simulink model "untitled"  (R2025b)
settings: Solver=VariableStepAuto  StartTime=0.0  StopTime=10.0  RelTol=1e-3
undefined symbols (not defined in the file): DiscIntNeverNeededParam
libraries: simulink x4
settings Model: Creator=mefe  LastModifiedBy=mefe

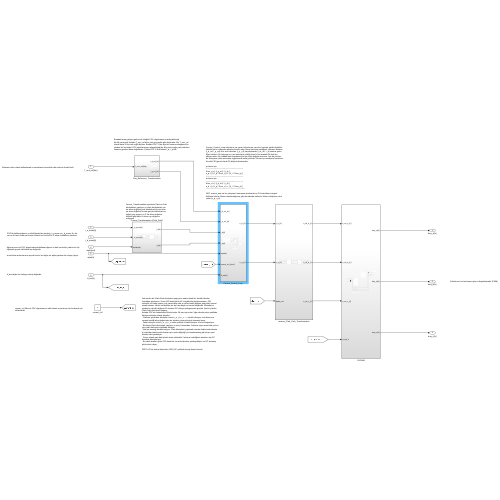
[thumbnail: Simulink's stored preview of the top-level diagram]
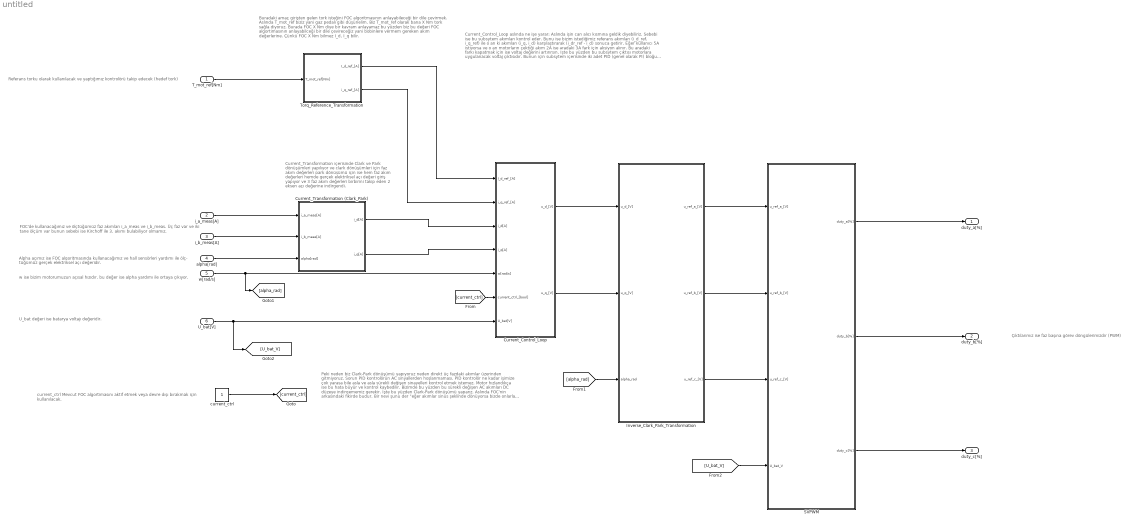
== system untitled ==
  note: Peki neden biz Clark-Park dönüşümü yapıyoruz neden direkt üç fazdaki akımlar üzerinden gitmiyoruz. Sorun PID kontrolörün AC sinyallerden hoşlanmaması. PID kontrolör ne kadar işimize çok yarasa bile asla ve asla sürekli değişen sinayelleri kontrol etmek istemez. Motor hızlandıkça ise bu hata büyür ve kontrol kaybedilir. Bizimde bu yüzden bu sürekli değişen AC akımları DC düzeye indirgememiz gerekir. İşte bu yüzden Clark-Park dönüşümü yaparız.
      | Aslında FOC'nin arkasındaki fikirde budur. Bir nevi şunu der "eğer akımlar sinüs şeklinde dönüyorsa bizde onlarla dönelim".
      | - Statorun gözünden dönüşüm öncesi i_a, i_b, i_c ---> sürekli dönüyor ve kullanıcının vermek istediği akım değerinden bu akımları çıkarıp kontrol etmemiz lazım.
      | - Fakat olmuyor çünkü i_a, i_b, i_c sinüs şeklinde sürekli dönüyor. Kontrol kayboluyor.
      | - İlk olarak Clark dönüşümü yapılıyor ve olay 3 eksenden 2 eksene iniyor ama hala çözüm yok çünkü hala sinüs şeklinde dönüyor.
      | - İşte işin mantığı burada başlıyor. Park dönüşümü yapılarak rotordan bakılıncaki akımlar ile statordan bakılıncaki akımlar aynı anda değiştiği için hareketsizmiş gibi oluyor yani akımlar sabit görünüyor.
      | - Sonuç olarak park dönüşümü sinüs şeklindeki 2 eksene indirdiğimiz akımları alıp DC akımlara dönüştürüyor.
      | - Bu sabit akımları gören PID kontrolör ise artık akımları yakalayabiliyor ve DC akımmış gibi kontrol ediyor.
      |
      | ÖZET: AC bir sistemi kontrolöre (PID) DC şeklinde tanıtıp kontrol etmek.
  note: Current_Control_Loop aslında ne işe yarar: Aslında işin can alıcı kısmına geldik diyebiliriz. Sebebi ise bu subsytem akımları kontrol eder. Bunu ise bizim istediğimiz referans akımları (i_d_ref, i_q_ref) ile o an ki akımları (i_q, i_d) karşılaştırarak (i_dr_ref - i_d) sonuca getirir. Eğer kullanıcı 5A istiyorsa ve o an motorların çektiği akım 2A ise aradaki 3A fark için aksiyon alınır. Bu aradaki farkı kapatmak için ise voltaj değerini artırırsın. İşte bu yüzden bu subsytem çıktısı motorlara uygulanacak voltaj çıktısıdır. Bunun için subsytem içerisinde iki adet PID (genel olarak PI) bloğu kullanılacaktır.
      |
      | q ekseni için
      | ----------------------------------------------------------
      | Error_q = [ (i_q_ref) - (i_q) ]
      | u_q = [ ( K_p * Error_q ) + ( K_i * Error_q ) ]
      | ----------------------------------------------------------
      | d ekseni için
      | ----------------------------------------------------------
      | Error_d = [ (i_d_ref) - (i_d) ]
      | u_d = [ ( K_p * Error_d ) + ( K_i * Error_d ) ]
      | -------------------------------------------------------------
      |
      | NOT: current_ena ise bu subsytem'i tamamen durdurmak ve PI kontrolünün integral birikimini sıfırlar. Motoru durdurduğumuz gibi durumlarda kullanılır. Motor voltajlarını sıfıra çeker (u_q, u_d).
  note: Buradaki amaç girişten gelen tork isteğini FOC algoritmasının anlayabileceği
      | bir dile çevirmek. Aslında T_mot_ref biziz yani gaz pedalı gibi düşünelim. Biz T_mot_ref olarak bana X Nm tork sağla diyoruz. Burada FOC X Nm diye bir kavram anlayamaz bu yüzden biz bu değeri FOC algortimasının anlayabilceği bir dile çevireceğiz yani bobinlere vermem gereken akım değerlerine. Çünkü FOC X Nm bilmez I_d, I_q bilir.
  note: Current_Transformation içerisinde Clark ve Park dönüşümleri yapılıyor ve clark dönüşümleri için faz akım değerleri park dönüşümü için ise hem faz akım değerleri hemde gerçek elektriksel açı değeri giriş yapıyor ve 3 faz akım değerleri birbirini takip eden 2 eksen açı değerine indirgendi.
  note: Çıktılarımız ise faz başına görev döngülerimizdir (PWM)
  note: U_bat değeri ise batarya voltajı değeridir.
  note: current_ctrl Mevcut FOC algortimasını aktif etmek veya devre dışı bırakmak için kullanılacak.
  note: w ise bizim motorumuzun açısal hızıdır. bu değer ise alpha yardımı ile ortaya çıkıyor.
  note: Alpha açımız ise FOC algoritmasında kullanacağımız ve hall sensörleri yardımı ile ölç-
      | tüğümüz gerçek elektriksel açı değeridir.
  note: FOC'de kullanacağımız ve ölçtüğümüz faz akımları i_a_meas ve i_b_meas. Üç faz var ve iki tane ölçüm var bunun sebebi ise Kirchoff ile 3. akımı bulabiliyor olmamız.
  note: Referans torku olarak kullanılacak ve yaptığımız kontrolörü takip edecek (hedef tork)
  T_mot_ref[Nm] : Inport
  i_a_meas[A] : Inport  Port=2
  i_b_meas[A] : Inport  Port=3
  alpha[rad] : Inport  Port=4
  w[rad/s] : Inport  Port=5
  U_bat[V] : Inport  Port=6
  Current_Control_Loop : Subsystem
  Current_Transformation (Clark_Park) : Subsystem
  Inverse_Clark_Park_Transformation : Subsystem
  SVPWM : Subsystem
  Torq_Reference_Transformation : Subsystem
  current_ctrl : Constant
  duty_a[%] : Outport
  duty_b[%] : Outport  Port=2
  duty_c[%] : Outport  Port=3
  wires:
  i_a_meas[A]/1 -> Current_Transformation (Clark_Park)/1(i_a_meas[A])
  i_b_meas[A]/1 -> Current_Transformation (Clark_Park)/2(i_b_meas[A])
  alpha[rad]/1 -> Current_Transformation (Clark_Park)/3(alpha[rad])
  T_mot_ref[Nm]/1 -> Torq_Reference_Transformation/1(T_mot_ref[Nm])
  Torq_Reference_Transformation/1(I_d_ref_[A]) -> Current_Control_Loop/1(I_d_ref_[A])
  Torq_Reference_Transformation/2(i_q_ref_[A]) -> Current_Control_Loop/2(i_q_ref_[A])
  Current_Transformation (Clark_Park)/1(i_d[A]) -> Current_Control_Loop/3(i_d[A])
  Current_Transformation (Clark_Park)/2(i_q[A]) -> Current_Control_Loop/4(i_q[A])
  current_ctrl/1 -> [current_ctrl]
  [current_ctrl] -> Current_Control_Loop/6(current_ctrl_[bool])
  w[rad/s]/1 -> [alpha_rad], Current_Control_Loop/5(w[rad/s])
  U_bat[V]/1 -> [U_bat_V], Current_Control_Loop/7(U_bat[V])
  [alpha_rad] -> Inverse_Clark_Park_Transformation/3(alpha_rad)
  Current_Control_Loop/2(u_q_[V]) -> Inverse_Clark_Park_Transformation/2(u_q_[V])
  Current_Control_Loop/1(u_d_[V]) -> Inverse_Clark_Park_Transformation/1(u_d_[V])
  Inverse_Clark_Park_Transformation/1(u_ref_a_[V]) -> SVPWM/1(u_ref_a_[V])
  Inverse_Clark_Park_Transformation/2(u_ref_b_[V]) -> SVPWM/2(u_ref_b_[V])
  Inverse_Clark_Park_Transformation/3(u_ref_c_[V]) -> SVPWM/3(u_ref_c_[V])
  [U_bat_V] -> SVPWM/4(U_bat_V)
  SVPWM/1(duty_a[%]) -> duty_a[%]/1
  SVPWM/3(duty_c[%]) -> duty_c[%]/1
  SVPWM/2(duty_b[%]) -> duty_b[%]/1

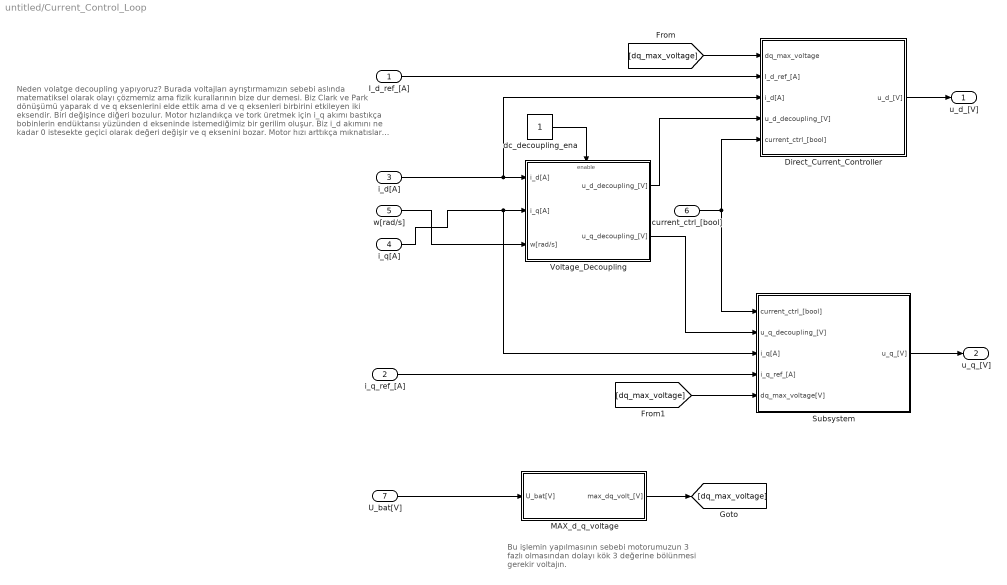
== system untitled/Current_Control_Loop ==
  note: Neden volatge decoupling yapıyoruz? Burada voltajları ayrıştırmamızın sebebi aslında matematiksel olarak olayı çözmemiz ama fizik kurallarının bize dur demesi. Biz Clark ve Park dönüşümü yaparak d ve q eksenlerini elde ettik ama d ve q eksenleri birbirini etkileyen iki eksendir. Biri değişince diğeri bozulur.
      | Motor hızlandıkça ve tork üretmek için i_q akımı bastıkça bobinlerin endüktansı yüzünden d ekseninde istemediğimiz bir gerilim oluşur.
      | Biz i_d akımını ne kadar 0 istesekte geçici olarak değeri değişir ve q eksenini bozar.
      | Motor hızı arttıkça mıknatıslar bobinlerde ters gerilim (Back-EMF) üretir. Bu gerilim doğrudan q eksenindeki voltajı düşürür.
      | NOT: Motor hızlandıkça torkun düşmesinin ana sebebi budur.
      | Peki bu olayların bu yapıya etkisi ne olur?
      | Yapı i_d =0 olsun ister. d ekseni PI kontrolcüsü işini yapmaya çalışır.
      | Yandan kullanıcı gaza basar yani i_q'yu arttırır ve fizik kuralları gereği d ekseninde bir dalgalanma olur.
      | Bu durumda PI kontrolcüsü bu hatayı düzeltmeye çalışır ama gecikmeli tepki verir ve kontrolden çıkar.
      |
      | NOT: FOC dögüsünden çıkıp yüksek hızlara giderken (Back-EMF) bu yapı hayat kurtaracak ve prüzsüz geçiş için yardımcı olacak.
  note: Bu işlemin yapılmasının sebebi motorumuzun
      | 3 fazlı olmasından dolayı kök 3 değerine
      | bölünmesi gerekir voltajın.
  I_d_ref_[A] : Inport
  i_q_ref_[A] : Inport  Port=2
  i_d[A] : Inport  Port=3
  i_q[A] : Inport  Port=4
  w[rad/s] : Inport  Port=5
  current_ctrl_[bool] : Inport  Port=6
  U_bat[V] : Inport  Port=7
  Direct_Current_Controller : Subsystem
  MAX_d_q_voltage : Subsystem
  Subsystem : Subsystem
  Voltage_Decoupling : Subsystem
  dc_decoupling_ena : Constant
  u_d_[V] : Outport
  u_q_[V] : Outport  Port=2
  wires:
  w[rad/s]/1 -> Voltage_Decoupling/3(w[rad/s])
  i_d[A]/1 -> Voltage_Decoupling/1(i_d[A]), Direct_Current_Controller/3(i_d[A])
  i_q[A]/1 -> Subsystem/3(i_q[A]), Voltage_Decoupling/2(i_q[A])
  I_d_ref_[A]/1 -> Direct_Current_Controller/2(I_d_ref_[A])
  Voltage_Decoupling/1(u_d_decoupling_[V]) -> Direct_Current_Controller/4(u_d_decoupling_[V])
  Direct_Current_Controller/1(u_d_[V]) -> u_d_[V]/1
  current_ctrl_[bool]/1 -> Subsystem/1(current_ctrl_[bool]), Direct_Current_Controller/5(current_ctrl_[bool])
  U_bat[V]/1 -> MAX_d_q_voltage/1(U_bat[V])
  MAX_d_q_voltage/1(max_dq_volt_[V]) -> [dq_max_voltage]
  [dq_max_voltage] -> Direct_Current_Controller/1(dq_max_voltage)
  Subsystem/1(u_q_[V]) -> u_q_[V]/1
  Voltage_Decoupling/2(u_q_decoupling_[V]) -> Subsystem/2(u_q_decoupling_[V])
  i_q_ref_[A]/1 -> Subsystem/4(i_q_ref_[A])
  [dq_max_voltage] -> Subsystem/5(dq_max_voltage[V])
  dc_decoupling_ena/1 -> Voltage_Decoupling/Enable

== system untitled/Current_Transformation (Clark_Park) ==
  i_a_meas[A] : Inport
  i_b_meas[A] : Inport  Port=2
  alpha[rad] : Inport  Port=3
  Clark_Transformation : Subsystem
  Park_Transformation : Subsystem
  i_d[A] : Outport
  i_q[A] : Outport  Port=2
  wires:
  i_a_meas[A]/1 -> Clark_Transformation/1(i_a_meas[A])
  i_b_meas[A]/1 -> Clark_Transformation/2(i_b_meas[A])
  Clark_Transformation/1(i_x[A]) -> Park_Transformation/1(i_x[A])  "i_x_meas"
  Clark_Transformation/2(i_y[A]) -> Park_Transformation/2(i_y[A])  "i_y_meas"
  alpha[rad]/1 -> Park_Transformation/3(alpha[rad])
  Park_Transformation/1(i_d[A]) -> i_d[A]/1  "i_d_meas"
  Park_Transformation/2(i_q[A]) -> i_q[A]/1  "i_q_meas"

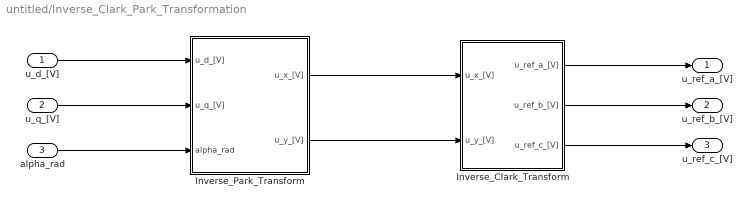
== system untitled/Inverse_Clark_Park_Transformation ==
  u_d_[V] : Inport
  u_q_[V] : Inport  Port=2
  alpha_rad : Inport  Port=3
  Inverse_Clark_Transform : Subsystem
  Inverse_Park_Transform : Subsystem
  u_ref_a_[V] : Outport
  u_ref_b_[V] : Outport  Port=2
  u_ref_c_[V] : Outport  Port=3
  wires:
  u_d_[V]/1 -> Inverse_Park_Transform/1(u_d_[V])
  u_q_[V]/1 -> Inverse_Park_Transform/2(u_q_[V])
  alpha_rad/1 -> Inverse_Park_Transform/3(alpha_rad)
  Inverse_Clark_Transform/1(u_ref_a_[V]) -> u_ref_a_[V]/1
  Inverse_Clark_Transform/3(u_ref_c_[V]) -> u_ref_c_[V]/1
  Inverse_Clark_Transform/2(u_ref_b_[V]) -> u_ref_b_[V]/1
  Inverse_Park_Transform/1(u_x_[V]) -> Inverse_Clark_Transform/1(u_x_[V])
  Inverse_Park_Transform/2(u_y_[V]) -> Inverse_Clark_Transform/2(u_y_[V])

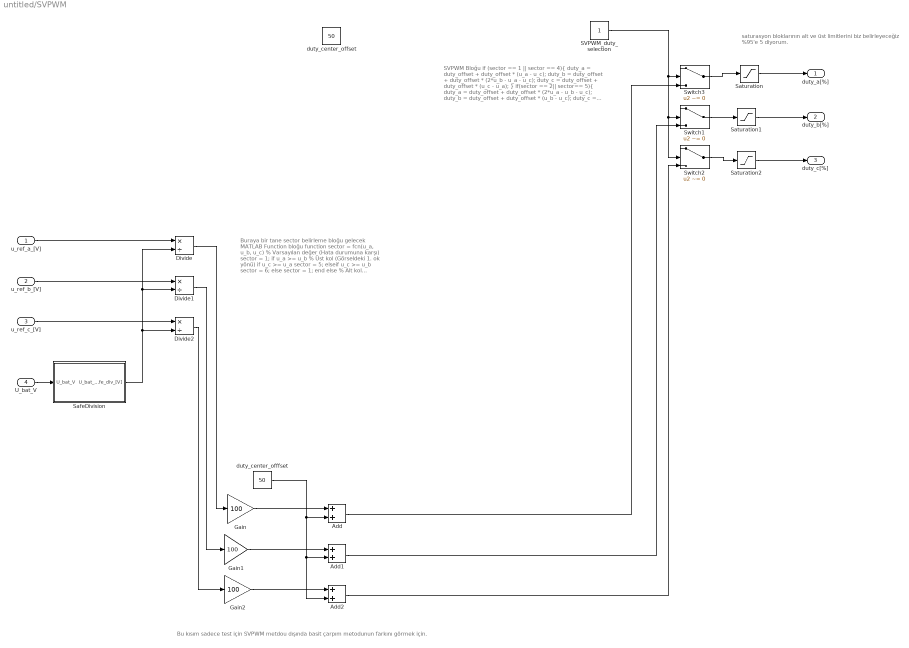
== system untitled/SVPWM ==
  note: saturasyon bloklarının alt ve üst limitlerini biz belirleyeceğiz
      | %95'e 5 diyorum.
  note: Bu kısım sadece test için SVPWM metdou dışında basit çarpım metodunun farkını görmek için.
  note: SVPWM Bloğu
      |
      | if (sector == 1 || sector == 4){
      | duty_a = duty_offset + duty_offset * (u_a - u_c);
      | duty_b = duty_offset + duty_offset * (2*u_b - u_a - u_c);
      | duty_c = duty_offset + duty_offset * (u_c - u_a);
      | }
      | if(sector == 2|| sector== 5){
      | duty_a = duty_offset + duty_offset * (2*u_a - u_b - u_c);
      | duty_b = duty_offset + duty_offset * (u_b - u_c);
      | duty_c = duty_offset + duty_offset * (u_c - u_b);
      | }
      | if(sector == 3 || sector == 6){
      | duty_c = duty_offset + duty_offset * (u_a - u_b);
      | duty_c = duty_offset + duty_offset * (u_b - u_a);
      | duty_a = duty_offset + duty_offset * (2*u_c - u_a - u_b);
      | }
  note: Buraya bir tane sector belirleme
      | bloğu gelecek
      | MATLAB Function bloğu
      | function sector = fcn(u_a, u_b, u_c)
      |     % Varsayılan değer (Hata durumuna karşı)
      |     sector = 1;
      |
      |     if u_a >= u_b
      |         % Üst kol (Görseldeki 1. ok yönü)
      |         if u_c >= u_a
      |             sector = 5;
      |         elseif u_c >= u_b
      |             sector = 6;
      |         else
      |             sector = 1;
      |         end
      |     else
      |         % Alt kol (Görseldeki 2. ok yönü: u_a < u_b)
      |         if u_c >= u_b
      |             sector = 2;
      |         elseif u_a >= u_c
      |             sector = 3;
      |         else
      |             sector = 4;
      |         end
      |     end
      | end
  u_ref_a_[V] : Inport
  u_ref_b_[V] : Inport  Port=2
  u_ref_c_[V] : Inport  Port=3
  U_bat_V : Inport  Port=4
  Add : Sum
  Add1 : Sum
  Add2 : Sum
  Divide : Product  Inputs=*/
  Divide1 : Product  Inputs=*/
  Divide2 : Product  Inputs=*/
  Gain : Gain  Gain=100  OutDataTypeStr=single
  Gain1 : Gain  Gain=100  OutDataTypeStr=single
  Gain2 : Gain  Gain=100  OutDataTypeStr=single
  SVPWM_duty_selection : Constant  OutDataTypeStr=boolean
  SafeDivision : Subsystem
  Saturation : Saturate  UpperLimit=95  LowerLimit=5
  Saturation1 : Saturate  UpperLimit=95  LowerLimit=5
  Saturation2 : Saturate  UpperLimit=95  LowerLimit=5
  Switch1 : Switch  Criteria=u2 ~= 0  SaturateOnIntegerOverflow=off  InputSameDT=off
  Switch2 : Switch  Criteria=u2 ~= 0  SaturateOnIntegerOverflow=off  InputSameDT=off
  Switch3 : Switch  Criteria=u2 ~= 0  SaturateOnIntegerOverflow=off  InputSameDT=off
  duty_center_offfset : Constant  Value=50  OutDataTypeStr=single
  duty_center_offset : Constant  Value=50  OutDataTypeStr=single
  duty_a[%] : Outport
  duty_b[%] : Outport  Port=2
  duty_c[%] : Outport  Port=3
  wires:
  U_bat_V/1 -> SafeDivision/1(U_bat_V)
  u_ref_b_[V]/1 -> Divide1/1
  u_ref_a_[V]/1 -> Divide/1
  u_ref_c_[V]/1 -> Divide2/1
  SafeDivision/1(U_bat_safe_div_[V]) -> Divide2/2, Divide1/2, Divide/2
  Gain/1 -> Add/1
  Gain1/1 -> Add1/1
  Gain2/1 -> Add2/1
  Divide2/1 -> Gain2/1
  Divide1/1 -> Gain1/1
  Divide/1 -> Gain/1
  duty_center_offfset/1 -> Add/2, Add2/2, Add1/2
  Add/1 -> Switch3/3
  Add1/1 -> Switch1/3
  Add2/1 -> Switch2/3
  SVPWM_duty_selection/1 -> Switch3/2, Switch1/2, Switch2/2
  Switch3/1 -> Saturation/1
  Switch1/1 -> Saturation1/1
  Switch2/1 -> Saturation2/1
  Saturation2/1 -> duty_c[%]/1
  Saturation1/1 -> duty_b[%]/1
  Saturation/1 -> duty_a[%]/1

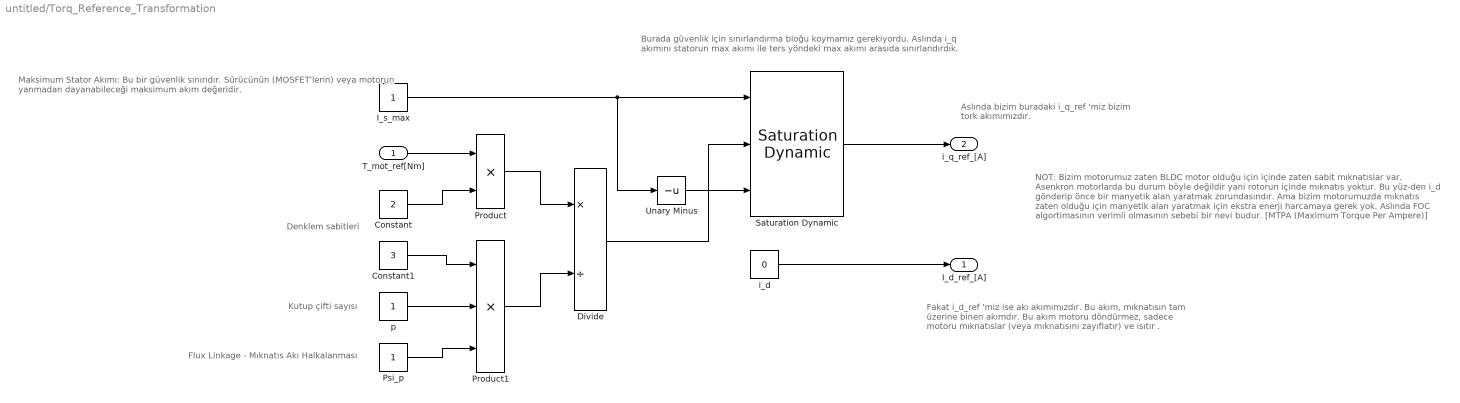
== system untitled/Torq_Reference_Transformation ==
  note: NOT: Bizim motorumuz zaten BLDC motor olduğu için içinde zaten sabit mıknatıslar var.
      | Asenkron motorlarda bu durum böyle değildir yani rotorun içinde mıknatıs yoktur. Bu yüz-den i_d gönderip önce bir manyetik alan yaratmak zorundasındır.
      | Ama bizim motorumuzda mıknatıs zaten olduğu için manyetik alan yaratmak için ekstra
      | enerji harcamaya gerek yok.
      | Aslında FOC algortimasının verimli olmasının sebebi bir nevi budur.
      | [MTPA (Maximum Torque Per Ampere)]
  note: Fakat i_d_ref 'miz ise akı akımımızdır.
      | Bu akım, mıknatısın tam üzerine binen akımdır.
      | Bu akım motoru döndürmez, sadece motoru mıknatıslar
      | (veya mıknatısını zayıflatır) ve ısıtır .
  note: Aslında bizim buradaki i_q_ref 'miz bizim
      | tork akımımızdır.
  note: Denklem sabitleri
  note: Burada güvenlik için sınırlandırma bloğu koymamız gerekiyordu. Aslında i_q
      | akımını statorun max akımı ile ters yöndeki max akımı arasıda sınırlandırdık.
  note: Maksimum Stator Akımı: Bu bir güvenlik sınırıdır. Sürücünün (MOSFET'lerin) veya motorun yanmadan dayanabileceği maksimum akım değeridir.
  note: Flux Linkage - Mıknatıs Akı Halkalanması
  note: Kutup çifti sayısı
  T_mot_ref[Nm] : Inport
  Constant : Constant  Value=2  OutDataTypeStr=single
  Constant1 : Constant  Value=3  OutDataTypeStr=single
  Divide : Product  Inputs=*/
  I_s_max : Constant
  Product : Product
  Product1 : Product  Inputs=3
  Psi_p : Constant
  Saturation Dynamic : simulink/Discontinuities/Saturation Dynamic  OutMin=[]  OutMax=[]  OutDataTypeStr=Inherit: Same as second input  OutDataType=fixdt(1, 16)  OutScaling=2^-10  DoSatur=off
  Unary Minus : UnaryMinus
  i_d : Constant  Value=0  OutDataTypeStr=single
  p : Constant
  I_d_ref_[A] : Outport
  i_q_ref_[A] : Outport  Port=2
  wires:
  T_mot_ref[Nm]/1 -> Product/1
  Constant/1 -> Product/2
  Constant1/1 -> Product1/1
  p/1 -> Product1/2
  Psi_p/1 -> Product1/3
  Product/1 -> Divide/1
  Product1/1 -> Divide/2
  I_s_max/1 -> Unary Minus/1, Saturation Dynamic/1
  Unary Minus/1 -> Saturation Dynamic/3
  Divide/1 -> Saturation Dynamic/2
  Saturation Dynamic/1 -> i_q_ref_[A]/1
  i_d/1 -> I_d_ref_[A]/1

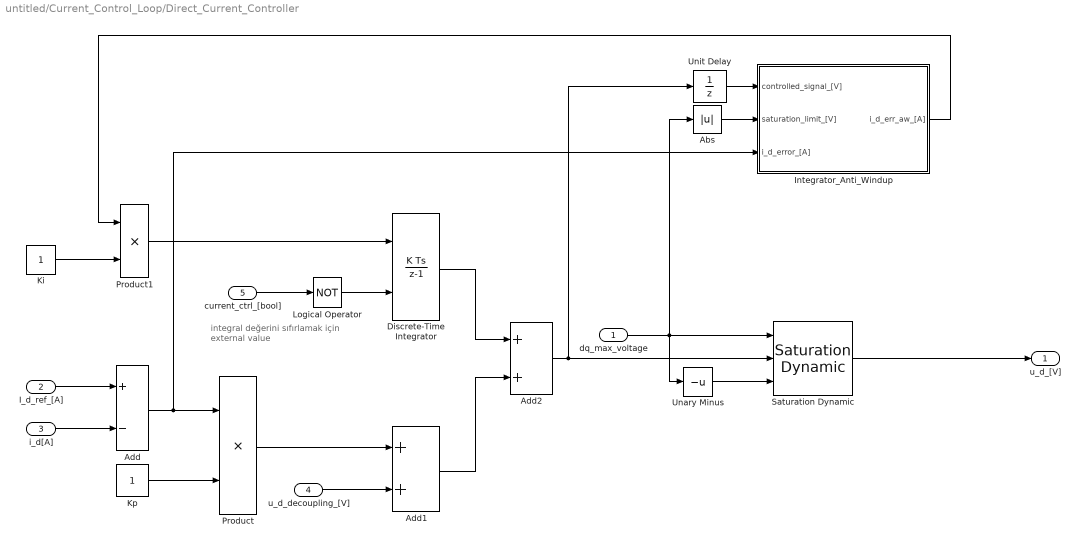
== system untitled/Current_Control_Loop/Direct_Current_Controller ==
  note: integral değerini
      | sıfırlamak için
      | external value
  dq_max_voltage : Inport
  I_d_ref_[A] : Inport  Port=2
  i_d[A] : Inport  Port=3
  u_d_decoupling_[V] : Inport  Port=4
  current_ctrl_[bool] : Inport  Port=5
  Abs : Abs  SaturateOnIntegerOverflow=off
  Add : Sum  Inputs=+-
  Add1 : Sum
  Add2 : Sum
  Discrete-Time Integrator : DiscreteIntegrator  ExternalReset=level  SampleTime=-1  ICPrevOutput=DiscIntNeverNeededParam  ICPrevScaledInput=DiscIntNeverNeededParam
  Integrator_Anti_Windup : Subsystem
  Ki : Constant
  Kp : Constant
  Logical Operator : Logic  Operator=NOT  AllPortsSameDT=off  OutDataTypeStr=boolean
  Product : Product
  Product1 : Product
  Saturation Dynamic : simulink/Discontinuities/Saturation Dynamic  OutMin=[]  OutMax=[]  OutDataTypeStr=Inherit: Same as second input  OutDataType=fixdt(1, 16)  OutScaling=2^-10  DoSatur=off
  Unary Minus : UnaryMinus
  Unit Delay : UnitDelay  SampleTime=-1  HasFrameUpgradeWarning=on
  u_d_[V] : Outport
  wires:
  I_d_ref_[A]/1 -> Add/1
  i_d[A]/1 -> Add/2
  Kp/1 -> Product/2
  Add/1 -> Integrator_Anti_Windup/3(i_d_error_[A]), Product/1
  Product/1 -> Add1/1
  u_d_decoupling_[V]/1 -> Add1/2
  Ki/1 -> Product1/2
  Product1/1 -> Discrete-Time Integrator/1
  current_ctrl_[bool]/1 -> Logical Operator/1
  Logical Operator/1 -> Discrete-Time Integrator/2
  Discrete-Time Integrator/1 -> Add2/1
  Add1/1 -> Add2/2
  Add2/1 -> Unit Delay/1, Saturation Dynamic/2
  Saturation Dynamic/1 -> u_d_[V]/1
  dq_max_voltage/1 -> Abs/1, Unary Minus/1, Saturation Dynamic/1
  Unary Minus/1 -> Saturation Dynamic/3
  Unit Delay/1 -> Integrator_Anti_Windup/1(controlled_signal_[V])
  Integrator_Anti_Windup/1(i_d_err_aw_[A]) -> Product1/1
  Abs/1 -> Integrator_Anti_Windup/2(saturation_limit_[V])

== system untitled/Current_Control_Loop/MAX_d_q_voltage ==
  U_bat[V] : Inport
  1/sqrt(3) (dq_voltage_ratio) : Constant
  Product : Product
  max_dq_volt_[V] : Outport
  wires:
  Product/1 -> max_dq_volt_[V]/1
  U_bat[V]/1 -> Product/1
  1/sqrt(3) (dq_voltage_ratio)/1 -> Product/2

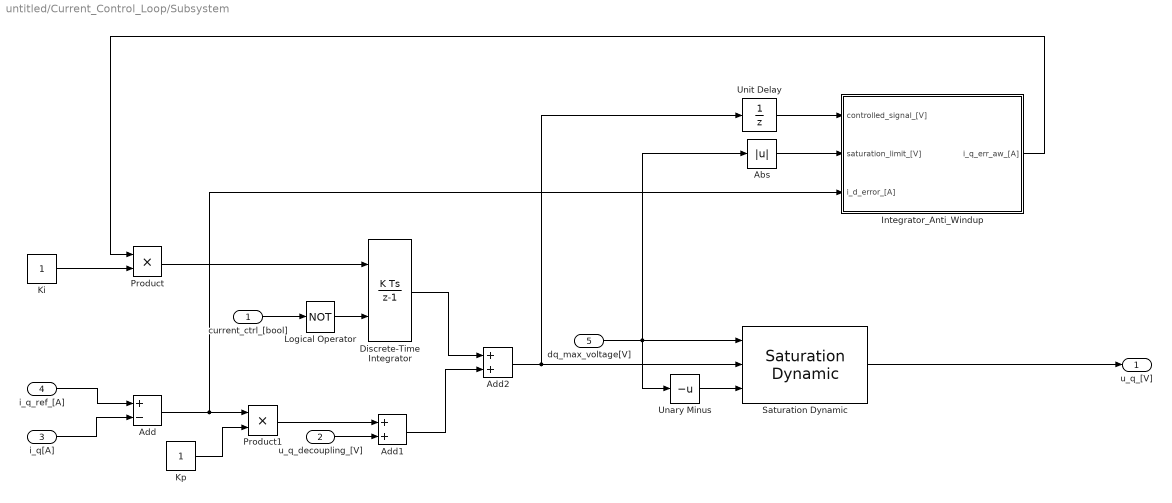
== system untitled/Current_Control_Loop/Subsystem ==
  current_ctrl_[bool] : Inport
  u_q_decoupling_[V] : Inport  Port=2
  i_q[A] : Inport  Port=3
  i_q_ref_[A] : Inport  Port=4
  dq_max_voltage[V] : Inport  Port=5
  Abs : Abs  SaturateOnIntegerOverflow=off
  Add : Sum  Inputs=+-
  Add1 : Sum
  Add2 : Sum
  Discrete-Time Integrator : DiscreteIntegrator  ExternalReset=level  SampleTime=-1  ICPrevOutput=DiscIntNeverNeededParam  ICPrevScaledInput=DiscIntNeverNeededParam
  Integrator_Anti_Windup : Subsystem
  Ki : Constant
  Kp : Constant
  Logical Operator : Logic  Operator=NOT  AllPortsSameDT=off  OutDataTypeStr=boolean
  Product : Product
  Product1 : Product
  Saturation Dynamic : simulink/Discontinuities/Saturation Dynamic  OutMin=[]  OutMax=[]  OutDataTypeStr=Inherit: Same as second input  OutDataType=fixdt(1, 16)  OutScaling=2^-10  DoSatur=off
  Unary Minus : UnaryMinus
  Unit Delay : UnitDelay  SampleTime=-1  HasFrameUpgradeWarning=on
  u_q_[V] : Outport
  wires:
  Unit Delay/1 -> Integrator_Anti_Windup/1(controlled_signal_[V])
  Abs/1 -> Integrator_Anti_Windup/2(saturation_limit_[V])
  Add/1 -> Integrator_Anti_Windup/3(i_d_error_[A]), Product1/1
  Integrator_Anti_Windup/1(i_q_err_aw_[A]) -> Product/1
  Ki/1 -> Product/2
  Kp/1 -> Product1/2
  i_q_ref_[A]/1 -> Add/1
  i_q[A]/1 -> Add/2
  Logical Operator/1 -> Discrete-Time Integrator/2
  current_ctrl_[bool]/1 -> Logical Operator/1
  Product/1 -> Discrete-Time Integrator/1
  Product1/1 -> Add1/1
  u_q_decoupling_[V]/1 -> Add1/2
  Discrete-Time Integrator/1 -> Add2/1
  Add1/1 -> Add2/2
  Add2/1 -> Saturation Dynamic/2, Unit Delay/1
  dq_max_voltage[V]/1 -> Abs/1, Unary Minus/1, Saturation Dynamic/1
  Unary Minus/1 -> Saturation Dynamic/3
  Saturation Dynamic/1 -> u_q_[V]/1

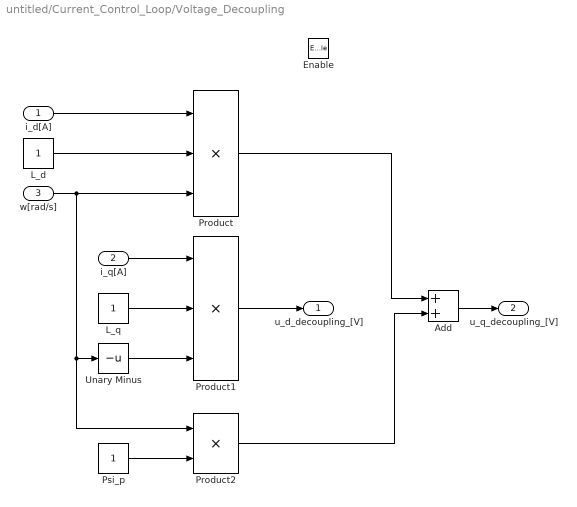
== system untitled/Current_Control_Loop/Voltage_Decoupling ==
  i_d[A] : Inport
  i_q[A] : Inport  Port=2
  w[rad/s] : Inport  Port=3
  Enable : EnablePort
  Add : Sum
  L_d : Constant
  L_q : Constant
  Product : Product  Inputs=3
  Product1 : Product  Inputs=3
  Product2 : Product
  Psi_p : Constant
  Unary Minus : UnaryMinus
  u_d_decoupling_[V] : Outport
  u_q_decoupling_[V] : Outport  Port=2
  wires:
  w[rad/s]/1 -> Product/3, Product2/1, Unary Minus/1
  i_d[A]/1 -> Product/1
  i_q[A]/1 -> Product1/1
  L_q/1 -> Product1/2
  Unary Minus/1 -> Product1/3
  L_d/1 -> Product/2
  Psi_p/1 -> Product2/2
  Product1/1 -> u_d_decoupling_[V]/1
  Product/1 -> Add/1
  Product2/1 -> Add/2
  Add/1 -> u_q_decoupling_[V]/1

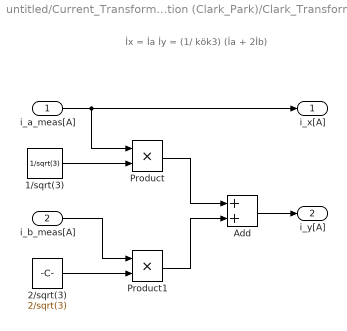
== system untitled/Current_Transformation (Clark_Park)/Clark_Transformation ==
  note: İx = İa
      |
      | İy = (1/ kök3) (İa + 2İb)
  i_a_meas[A] : Inport
  i_b_meas[A] : Inport  Port=2
  1/sqrt(3) : Constant  Value=1/sqrt(3)  OutDataTypeStr=single
  2/sqrt(3) : Constant  Value=2/sqrt(3)  OutDataTypeStr=single
  Add : Sum
  Product : Product
  Product1 : Product
  i_x[A] : Outport
  i_y[A] : Outport  Port=2
  wires:
  i_a_meas[A]/1 -> Product/1, i_x[A]/1
  1/sqrt(3)/1 -> Product/2
  i_b_meas[A]/1 -> Product1/1
  2/sqrt(3)/1 -> Product1/2
  Product/1 -> Add/1
  Product1/1 -> Add/2
  Add/1 -> i_y[A]/1

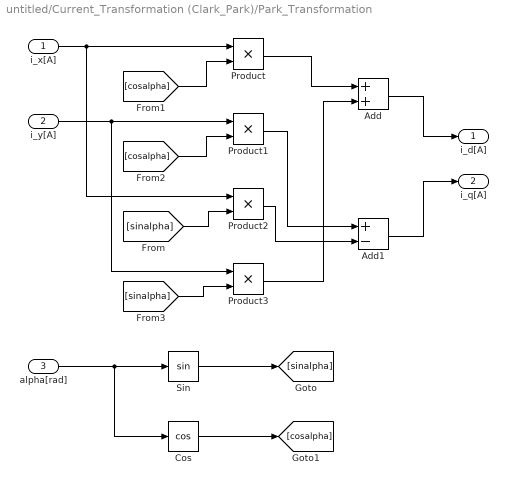
== system untitled/Current_Transformation (Clark_Park)/Park_Transformation ==
  i_x[A] : Inport
  i_y[A] : Inport  Port=2
  alpha[rad] : Inport  Port=3
  Add : Sum
  Add1 : Sum  Inputs=+-
  Cos : Trigonometry  Operator=cos
  Product{,1..3} (4 alike) : Product
  Sin : Trigonometry
  i_d[A] : Outport
  i_q[A] : Outport  Port=2
  wires:
  alpha[rad]/1 -> Sin/1, Cos/1
  Sin/1 -> [sinalpha]
  Cos/1 -> [cosalpha]
  i_x[A]/1 -> Product/1, Product2/1
  i_y[A]/1 -> Product1/1, Product3/1
  [cosalpha] -> Product/2
  [sinalpha] -> Product3/2
  Product/1 -> Add/1
  Add/1 -> i_d[A]/1
  Add1/1 -> i_q[A]/1
  [sinalpha] -> Product2/2
  [cosalpha] -> Product1/2
  Product1/1 -> Add1/1
  Product3/1 -> Add/2
  Product2/1 -> Add1/2

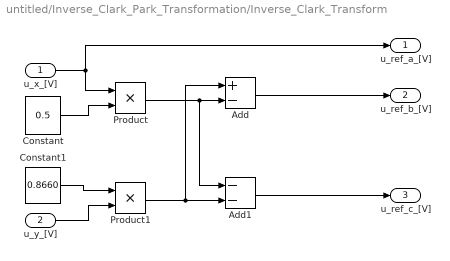
== system untitled/Inverse_Clark_Park_Transformation/Inverse_Clark_Transform ==
  u_x_[V] : Inport
  u_y_[V] : Inport  Port=2
  Add : Sum  Inputs=+-
  Add1 : Sum  Inputs=--
  Constant : Constant  Value=0.5
  Constant1 : Constant  Value=0.8660
  Product : Product
  Product1 : Product
  u_ref_a_[V] : Outport
  u_ref_b_[V] : Outport  Port=2
  u_ref_c_[V] : Outport  Port=3
  wires:
  u_x_[V]/1 -> u_ref_a_[V]/1, Product/1
  Constant/1 -> Product/2
  Constant1/1 -> Product1/1
  u_y_[V]/1 -> Product1/2
  Product/1 -> Add1/1, Add/2
  Product1/1 -> Add1/2, Add/1
  Add/1 -> u_ref_b_[V]/1
  Add1/1 -> u_ref_c_[V]/1

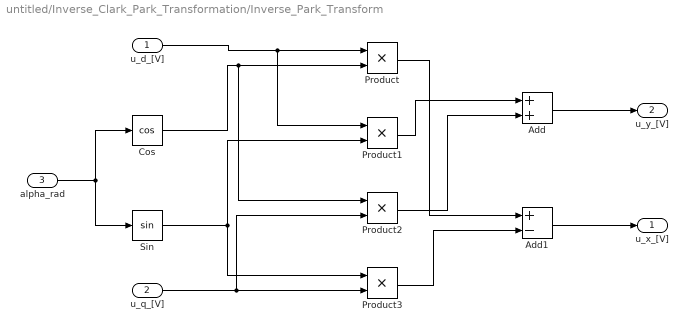
== system untitled/Inverse_Clark_Park_Transformation/Inverse_Park_Transform ==
  u_d_[V] : Inport
  u_q_[V] : Inport  Port=2
  alpha_rad : Inport  Port=3
  Add : Sum
  Add1 : Sum  Inputs=+-
  Cos : Trigonometry  Operator=cos
  Product{,1..3} (4 alike) : Product
  Sin : Trigonometry
  u_x_[V] : Outport
  u_y_[V] : Outport  Port=2
  wires:
  alpha_rad/1 -> Cos/1, Sin/1
  u_d_[V]/1 -> Product1/1, Product/1
  Cos/1 -> Product/2, Product2/1
  Sin/1 -> Product3/1, Product1/2
  u_q_[V]/1 -> Product2/2, Product3/2
  Product3/1 -> Add1/2
  Product/1 -> Add1/1
  Product1/1 -> Add/1
  Product2/1 -> Add/2
  Add1/1 -> u_x_[V]/1
  Add/1 -> u_y_[V]/1

== system untitled/SVPWM/SafeDivision ==
  U_bat_V : Inport
  Compare To Constant : simulink/Logic and Bit Operations/Compare To Constant  relop===  const=0.0  OutDataTypeStr=boolean
  Constant : Constant  Value=1e-6
  Switch : Switch  Criteria=u2 ~= 0  SaturateOnIntegerOverflow=off  InputSameDT=off
  U_bat_safe_div_[V] : Outport
  wires:
  Constant/1 -> Switch/1
  Compare To Constant/1 -> Switch/2
  U_bat_V/1 -> Compare To Constant/1, Switch/3
  Switch/1 -> U_bat_safe_div_[V]/1

== system untitled/Current_Control_Loop/Direct_Current_Controller/Integrator_Anti_Windup ==
  controlled_signal_[V] : Inport
  saturation_limit_[V] : Inport  Port=2
  i_d_error_[A] : Inport  Port=3
  Abs : Abs  SaturateOnIntegerOverflow=off
  Product : Product
  Relational Operator : RelationalOperator  Operator=<  OutDataTypeStr=boolean  RndMeth=Simplest  InputSameDT=off
  i_d_err_aw_[A] : Outport
  wires:
  controlled_signal_[V]/1 -> Abs/1
  Abs/1 -> Relational Operator/1
  saturation_limit_[V]/1 -> Relational Operator/2
  i_d_error_[A]/1 -> Product/2
  Relational Operator/1 -> Product/1
  Product/1 -> i_d_err_aw_[A]/1

== system untitled/Current_Control_Loop/Subsystem/Integrator_Anti_Windup ==
  controlled_signal_[V] : Inport
  saturation_limit_[V] : Inport  Port=2
  i_d_error_[A] : Inport  Port=3
  Abs : Abs  SaturateOnIntegerOverflow=off
  Product : Product
  Relational Operator : RelationalOperator  Operator=<  OutDataTypeStr=boolean  RndMeth=Simplest  InputSameDT=off
  i_q_err_aw_[A] : Outport
  wires:
  saturation_limit_[V]/1 -> Relational Operator/2
  Abs/1 -> Relational Operator/1
  controlled_signal_[V]/1 -> Abs/1
  i_d_error_[A]/1 -> Product/2
  Relational Operator/1 -> Product/1
  Product/1 -> i_q_err_aw_[A]/1
